simulink model "magnet"  (Simulink 7.3)
settings: Solver=ode3  StartTime=0.0  StopTime=100.0  FixedStep=0.01  RelTol=1e-3
undefined symbols (not defined in the file or in its folder): magnet_force
libraries: simulink x1
settings Model: Creator=psoltysiak  LastModifiedBy=psoltysiak

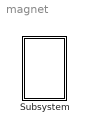
== system magnet ==
  Subsystem : Subsystem  mask{k=0.3, l=5, m=4, startX=2, startY=1.74, g=9.81}
      mask prompts: k "hamowanie"; l "dlugosc"; m "masa"; startX "pocz- X kulki"; startY "pocz Y kulki"; g "grawitacja"

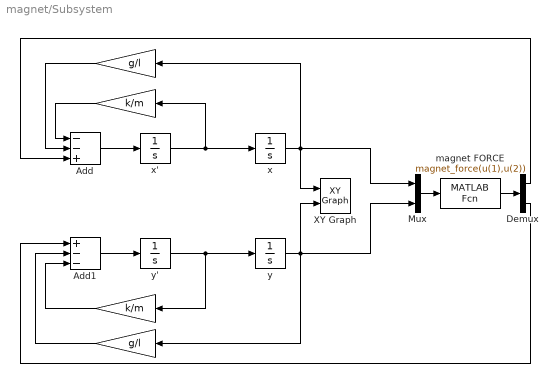
== system magnet/Subsystem ==
  " " : Gain  Gain=g/l  ParameterDataType=fixdt(1, 16)  ParameterScaling=2^0  OutDataType=fixdt(1, 16)  OutScaling=2^0
  "   " : Gain  Gain=k/m  ParameterDataType=fixdt(1, 16)  ParameterScaling=2^0  OutDataType=fixdt(1, 16)  OutScaling=2^0
  "    " : Gain  Gain=k/m  ParameterDataType=fixdt(1, 16)  ParameterScaling=2^0  OutDataType=fixdt(1, 16)  OutScaling=2^0
  "     " : Gain  Gain=g/l  ParameterDataType=fixdt(1, 16)  ParameterScaling=2^0  OutDataType=fixdt(1, 16)  OutScaling=2^0
  Add : Sum  Inputs=--+  OutDataType=fixdt(1, 16)  OutScaling=2^-10
  Add1 : Sum  Inputs=+--  OutDataType=fixdt(1, 16)  OutScaling=2^-10
  Demux : Demux  Outputs=2
  Mux : Mux  Inputs=2
  XY Graph : simulink/Sinks/XY Graph  SystemSampleTime=-1  xmin=-3  xmax=3  ymin=-3  ymax=3  st=-1
  magnet FORCE : MATLABFcn  MATLABFcn=magnet_force(u(1),u(2))
  x : Integrator  InitialCondition=startX
  x' : Integrator
  y : Integrator  InitialCondition=startY
  y' : Integrator
  wires:
  x'/1 -> x/1, "    "/1
  Add/1 -> x'/1
  "    "/1 -> Add/1
  x/1 -> "     "/1, XY Graph/1, Mux/1
  "     "/1 -> Add/2
  y'/1 -> "   "/1, y/1
  "   "/1 -> Add1/3
  " "/1 -> Add1/2
  Add1/1 -> y'/1
  y/1 -> Mux/2, XY Graph/2, " "/1
  Demux/2 -> Add1/1
  Demux/1 -> Add/3
  Mux/1 -> magnet FORCE/1
  magnet FORCE/1 -> Demux/1
